simulink model "Stewart"  (Simulink 7.0)
settings: Solver=ode1  StartTime=0.0  StopTime=inf  FixedStep=0.001  RelTol=1e-3
libraries: mblibv1 x50, quarc_library x1
settings Model: Creator=colinlea  LastModifiedBy=colinlea  ExtModeTrigDuration=10000
settings SolverCC: PositivePriorityOrder=on
settings RTWCC: SystemTargetFile=quarc_windows.tlc  TemplateMakefile=quarc_default_tmf  Description=QuaRC Win32 Target  ProcessScript=quarc_windows_make_rtw_hook
settings STFCustomTargetCC: TargetPreCompLibLocation=C:\DOCUME~1\ALLUSE~1\APPLIC~1\QuaRC\lib\2007b\windows\release  GenFloatMathFcnCalls=ANSI_C  SystemTargetFile=quarc_windows.tlc
settings GRTTargetCC: TargetPreCompLibLocation=C:\DOCUME~1\ALLUSE~1\APPLIC~1\QuaRC\lib\2007b\windows\release  CompOptLevelCompliant=off  MatFileLogging=off  ExtMode=on  ExtModeMexFile=quarc_comm
settings SimMechanicsCC: VisOnUpdateDiagram=on  VisDuringSimulation=on

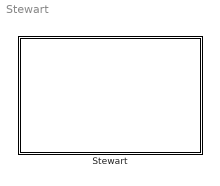
== system Stewart ==
  Stewart : Subsystem

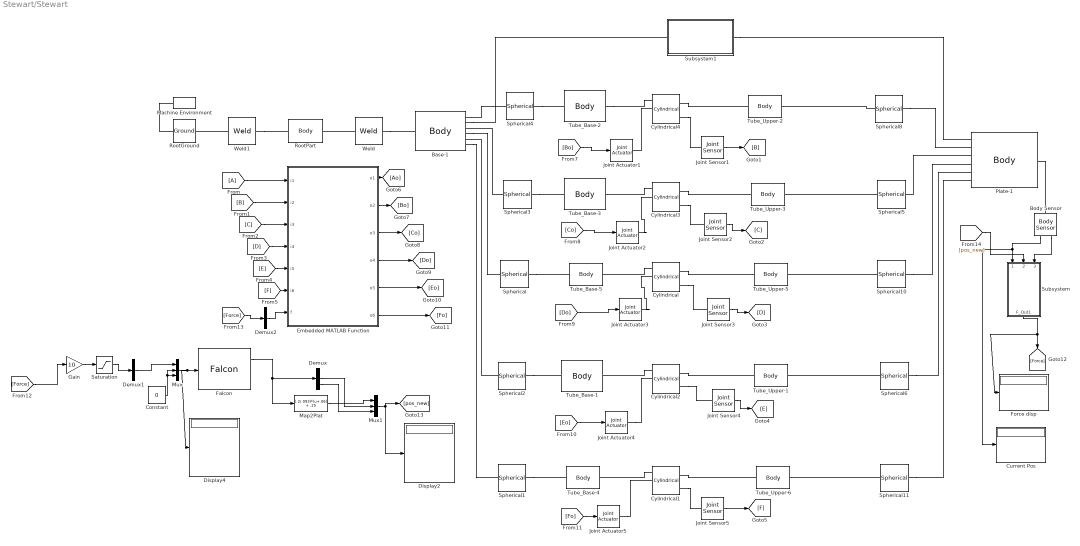
== system Stewart/Stewart ==
  Base-1 : mblibv1/Bodies/Body  DialogController=MECH.DynMechDlgSource  PhysicalDomain=mechanical  SubClassName=Unknown  LeftPortType=workingframe  RightPortType=workingframe  LConnTagsString=CS2  RConnTagsString=CS5|CS8|CS4|CS7|CS3|CS6  DialogClass=MechanicalBodyBlock  Mass=1.0825  MassUnits=kg  InertiaUnits=kg*m^2  Inertia=[0.011284 0 0;0 0.022551 0;0 0 0.011285]  Shape=Cylinder  ShapeDims=[1 1]  ShapeUnits=m  ShapeUse=false  Density=1  DensityUnits=kg/m^3  DensityUse=false  CG=Right$CG$[-0.030204 -0.023928 0.035595]$WORLD$WORLD$m$[1 0 0;0 1 0;0 0 1]$3x3 Transform$rad$WORLD$false  WorkingFrames=Right$CS5$[0.2198 -0.018929 -0.10874]$WORLD$WORLD$m$[1 0 0;0 1 0;0 0 1]$3x3 Transform$rad$WORLD$true#Right$CS8$[0.2198 -0.018929 -0.10874]$WORLD$WORLD$m$[1 0 0;0 1 0;0 0 1]$3x3 Transform$rad$WORLD$true#Left$CS2$[-0.030204 -0.023928 0.035595]$WORLD$WORLD$m$[1 0 0;0 1 0;0 0 1]$3x3 Transform$rad$WORLD$true#Right$CS4$[-0.2802 -0.018929 -0.10874]$WORLD$WORLD$m$[1 0 0;0 1 0;0 0 1]$3x3 Transform$rad$WORLD$true#Right$CS7$[-0.2802 -0.018929 -0.10874]$WORLD$WORLD$m$[1 0 0;0 1 0;0 0 1]$3x3 Transform$rad$WORLD$true#Right$CS3$[-0.030204 -0.018929 0.32426]$WORLD$WORLD$m$[1 0 0;0 1 0;0 0 1]$3x3 Transform$rad$WORLD$true#Right$CS6$[-0.030204 -0.018929 0.32426]$WORLD$WORLD$m$[1 0 0;0 1 0;0 0 1]$3x3 Transform$rad$WORLD$true#Right$CS1$[-0.030204 -0.028928 0.035592]$WORLD$WORLD$m$[1 0 0;0 1 0;0 0 1]$3x3 Transform$rad$WORLD$false  CGPos=[-0.030204 -0.023928 0.035595]  CGRot=[1 0 0;0 1 0;0 0 1]  CS0Pos=[]  CS0Rot=[]  CS1Pos=[-0.030204 -0.028928 0.035592]  CS1Rot=[1 0 0;0 1 0;0 0 1]  CS2Pos=[-0.030204 -0.023928 0.035595]  CS2Rot=[1 0 0;0 1 0;0 0 1]  CS3Pos=[-0.030204 -0.018929 0.32426]  CS3Rot=[1 0 0;0 1 0;0 0 1]  CS4Pos=[-0.2802 -0.018929 -0.10874]  CS4Rot=[1 0 0;0 1 0;0 0 1]  CS5Pos=[0.2198 -0.018929 -0.10874]  CS5Rot=[1 0 0;0 1 0;0 0 1]  CS6Pos=[-0.030204 -0.018929 0.32426]  CS6Rot=[1 0 0;0 1 0;0 0 1]  CS7Pos=[-0.2802 -0.018929 -0.10874]  CS7Rot=[1 0 0;0 1 0;0 0 1]  CS8Pos=[0.2198 -0.018929 -0.10874]  CS8Rot=[1 0 0;0 1 0;0 0 1]  CS9Pos=[]  CS9Rot=[]  CS10Pos=[]  CS10Rot=[]  CS11Pos=[]  CS11Rot=[]  CS12Pos=[]  CS12Rot=[]  CS13Pos=[]  CS13Rot=[]  CS14Pos=[]  CS14Rot=[]  CS15Pos=[]  CS15Rot=[]  CS16Pos=[]  CS16Rot=[]  CS17Pos=[]  CS17Rot=[]  CS18Pos=[]  CS18Rot=[]  CS19Pos=[]  CS19Rot=[]  CS20Pos=[]  CS20Rot=[]
  Body Sensor : mblibv1/Sensors &  Actuators/Body Sensor  Orientation=down  DialogController=MECH.DynMechDlgSource  SystemSampleTime=-1  PhysicalDomain=Mechanical  PortType=blob  Muxed=off  Pose=off  Angle=on  AngleUnits=deg  ArcVelocity=off  ArcVelocityUnits=deg/s  ArcAcceleration=off  ArcAccelerationUnits=deg/s^2  CoordPosition=on  CoordPositionUnits=m  Velocity=on  VelocityUnits=m/s  Acceleration=off  AccelerationUnits=m/s^2  Quaternion=on  QuaternionDT=off  QuaternionDDT=off  QuaternionUnits=off  OutputVector=[1]  ActiveIO=on  Width=6  DialogClass=MechanicalSensorBlock  ReferenceFrame=Absolute (World)
  Constant : Constant  Value=0  OutDataType=sfix(16)  OutScaling=2^0
  Current Pos : Display
  Cylindrical : mblibv1/Joints/Cylindrical  DialogController=MECH.DynMechDlgSource  PhysicalDomain=mechanical  SubClassName=Unknown  LeftPortType=blob  RightPortType=blob  LConnTagsString=__newl0|SA1|SA2  RConnTagsString=__newr0|SA1  NumSAPorts=3  CutJoint=off  MarkAsCut=off  Primitives=prismatic  PrimitiveProps=P1$World$[-0.28308 -0.90664 -0.31285]$prismatic#R1$World$[-0.28308 -0.90664 -0.31285]$revolute  DialogClass=JointBlock  P1Axis=[-0.28308 -0.90664 -0.31285]  R1Axis=[-0.28308 -0.90664 -0.31285]
  Cylindrical1 : mblibv1/Joints/Cylindrical  DialogController=MECH.DynMechDlgSource  PhysicalDomain=mechanical  SubClassName=Unknown  LeftPortType=blob  RightPortType=blob  LConnTagsString=__newl0|SA1|SA2  RConnTagsString=__newr0|SA1  NumSAPorts=3  CutJoint=off  MarkAsCut=off  Primitives=prismatic  PrimitiveProps=P1$World$[0.17265 -0.86638 0.46859]$prismatic#R1$World$[0.17265 -0.86638 0.46859]$revolute  DialogClass=JointBlock  P1Axis=[0.17265 -0.86638 0.46859]  R1Axis=[0.17265 -0.86638 0.46859]
  Cylindrical2 : mblibv1/Joints/Cylindrical  DialogController=MECH.DynMechDlgSource  PhysicalDomain=mechanical  SubClassName=Unknown  LeftPortType=blob  RightPortType=blob  LConnTagsString=__newl0|SA1|SA2  RConnTagsString=__newr0|SA1  NumSAPorts=3  CutJoint=off  MarkAsCut=off  Primitives=prismatic  PrimitiveProps=P1$World$[-0.24223 -0.7709 0.58909]$prismatic#R1$World$[-0.24223 -0.7709 0.58909]$revolute  DialogClass=JointBlock  P1Axis=[-0.24223 -0.7709 0.58909]  R1Axis=[-0.24223 -0.7709 0.58909]
  Cylindrical3 : mblibv1/Joints/Cylindrical  DialogController=MECH.DynMechDlgSource  PhysicalDomain=mechanical  SubClassName=Unknown  LeftPortType=blob  RightPortType=blob  LConnTagsString=__newl0|SA1|SA2  RConnTagsString=__newr0|SA1  NumSAPorts=3  CutJoint=off  MarkAsCut=off  Primitives=prismatic  PrimitiveProps=P1$World$[-0.42557 -0.8936 0.14272]$prismatic#R1$World$[-0.42557 -0.8936 0.14272]$revolute  DialogClass=JointBlock  P1Axis=[-0.42557 -0.8936 0.14272]  R1Axis=[-0.42557 -0.8936 0.14272]
  Cylindrical4 : mblibv1/Joints/Cylindrical  DialogController=MECH.DynMechDlgSource  PhysicalDomain=mechanical  SubClassName=Unknown  LeftPortType=blob  RightPortType=blob  LConnTagsString=__newl0|SA1|SA2  RConnTagsString=__newr0|SA1  NumSAPorts=3  CutJoint=off  MarkAsCut=off  Primitives=prismatic  PrimitiveProps=P1$World$[0.24469 -0.94526 -0.21591]$prismatic#R1$World$[0.24469 -0.94526 -0.21591]$revolute  DialogClass=JointBlock  P1Axis=[0.24469 -0.94526 -0.21591]  R1Axis=[0.24469 -0.94526 -0.21591]
  Demux : Demux  Outputs=3
  Demux1 : Demux  Outputs=3
  Demux2 : Demux  Outputs=3
  Display2 : Display
  Display4 : Display
  Embedded MATLAB Function : Stateflow chart
  Falcon : quarc_library/Devices/Third-Party/Novint/Falcon  sample_time=qc_get_step_size  show_calibrate=off
  Force disp : Display
  Gain : Gain  Gain=10  ParameterDataType=sfix(16)  ParameterScaling=2^0  OutDataType=sfix(16)  OutScaling=2^0
  Joint Actuator{1..5} (5 alike) : mblibv1/Sensors &  Actuators/Joint Actuator  DialogController=MECH.DynMechDlgSource  SystemSampleTime=-1  PhysicalDomain=Mechanical  PortType=blob  ActuationStyle=Force  AngleUnits=deg  ArcVelocityUnits=deg/s  ArcAccelerationUnits=deg/s^2  CoordPositionUnits=m  VelocityUnits=m/s  AccelerationUnits=m/s^2  ForceUnits=N  TorqueUnits=N*m  ActiveIO=on  Width=1  DialogClass=MechanicalActuatorBlock  Primitive=P1  ReferenceFrame=Absolute (World)
  Joint Sensor{1..5} (5 alike) : mblibv1/Sensors &  Actuators/Joint Sensor  DialogController=MECH.DynMechDlgSource  SystemSampleTime=-1  PhysicalDomain=Mechanical  PortType=blob  Muxed=on  Pose=off  Angle=on  AngleUnits=deg  ArcVelocity=off  ArcVelocityUnits=deg/s  ArcAcceleration=off  ArcAccelerationUnits=deg/s^2  CoordPosition=on  CoordPositionUnits=m  Velocity=off  VelocityUnits=m/s  Acceleration=off  AccelerationUnits=m/s^2  Quaternion=on  QuaternionDT=off  QuaternionDDT=off  QuaternionUnits=off  OutputVector=[1]  ActiveIO=on  Width=1  DialogClass=MechanicalSensorBlock  Primitive=P1  Force=off  ForceUnits=N  Torque=off  TorqueUnits=N-m  ReferenceFrame=Absolute (World)  ReactionSensedSide=Base  ReactionReferenceFrame=Absolute (World)  ReactionForce=off  ReactionForceUnits=N  ReactionMoment=off  ReactionMomentUnits=N-m
  Machine Environment : mblibv1/Bodies/Machine Environment  Orientation=left  DialogController=MECH.DialogSource  SystemSampleTime=-1  PortType=env  PhysicalDomain=Mechanical  DialogTemplateClass=MECH.MachineEnvironment  SyncWhenCopied=off  Gravity=[0 0 0]  GravityUnits=m/s^2  GravityAsSignal=off  Dimensionality=Auto-detect  AnalysisType=Forward dynamics  LinearAssemblyTolerance=1e-3  LinearAssemblyToleranceUnits=m  AngularAssemblyTolerance=1e-3  AngularAssemblyToleranceUnits=rad  ConstraintSolverType=Stabilizing  ConstraintRelTolerance=1e-4  ConstraintAbsTolerance=1e-4  UseRobustSingularityHandling=off  RedundancyAnalysisToleranceType=Automatically select tolerance  RedundancyAnalysisTolerance=1e-14  StatePerturbationType=Fixed  PerturbationSize=1e-5  VisualizeMachine=on
  Map2Plat : Fcn  Expr=(.2/.093)*(u+.06) + .25
  Mux : Mux  Inputs=3
  Mux1 : Mux  Inputs=3
  Plate-1 : mblibv1/Bodies/Body  DialogController=MECH.DynMechDlgSource  PhysicalDomain=mechanical  SubClassName=Unknown  LeftPortType=workingframe  RightPortType=workingframe  LConnTagsString=CS5|CS4|CS2|CS6|CS3|CS7  RConnTagsString=CG  DialogClass=MechanicalBodyBlock  Mass=0.27063  MassUnits=kg  InertiaUnits=kg*m^2  Inertia=[0.00070697 0 0;0 0.0014095 0;0 0 0.00070701]  Shape=Cylinder  ShapeDims=[1 1]  ShapeUnits=m  ShapeUse=false  Density=1  DensityUnits=kg/m^3  DensityUse=false  CG=Right$CG$[-0.032335 0.43541 -0.043031]$WORLD$WORLD$m$[0.19654 0.14624 0.96953;-0.26061 0.96104 -0.092126;-0.94523 -0.23456 0.227]$3x3 Transform$rad$WORLD$true  WorkingFrames=Left$CS5$[-0.078466 0.40468 -0.17639]$WORLD$WORLD$m$[1 0 0;0 1 0;0 0 1]$3x3 Transform$rad$WORLD$true#Left$CS4$[0.10687 0.41731 -0.0090952]$WORLD$WORLD$m$[1 0 0;0 1 0;0 0 1]$3x3 Transform$rad$WORLD$true#Left$CS2$[-0.078466 0.40468 -0.17639]$WORLD$WORLD$m$[1 0 0;0 1 0;0 0 1]$3x3 Transform$rad$WORLD$true#Left$CS6$[-0.1276 0.46983 0.059914]$WORLD$WORLD$m$[1 0 0;0 1 0;0 0 1]$3x3 Transform$rad$WORLD$true#Left$CS3$[0.10687 0.41731 -0.0090952]$WORLD$WORLD$m$[1 0 0;0 1 0;0 0 1]$3x3 Transform$rad$WORLD$true#Left$CS7$[-0.1276 0.46983 0.059914]$WORLD$WORLD$m$[1 0 0;0 1 0;0 0 1]$3x3 Transform$rad$WORLD$true#Right$CS1$[-0.033072 0.43061 -0.04186]$WORLD$WORLD$m$[0.19654 0.14624 0.96953;-0.26061 0.96104 -0.092126;-0.94523 -0.23456 0.227]$3x3 Transform$rad$WORLD$false  CGPos=[-0.032335 0.43541 -0.043031]  CGRot=[0.19654 0.14624 0.96953;-0.26061 0.96104 -0.092126;-0.94523 -0.23456 0.227]  CS0Pos=[]  CS0Rot=[]  CS1Pos=[-0.033072 0.43061 -0.04186]  CS1Rot=[0.19654 0.14624 0.96953;-0.26061 0.96104 -0.092126;-0.94523 -0.23456 0.227]  CS2Pos=[-0.078466 0.40468 -0.17639]  CS2Rot=[1 0 0;0 1 0;0 0 1]  CS3Pos=[0.10687 0.41731 -0.0090952]  CS3Rot=[1 0 0;0 1 0;0 0 1]  CS4Pos=[0.10687 0.41731 -0.0090952]  CS4Rot=[1 0 0;0 1 0;0 0 1]  CS5Pos=[-0.078466 0.40468 -0.17639]  CS5Rot=[1 0 0;0 1 0;0 0 1]  CS6Pos=[-0.1276 0.46983 0.059914]  CS6Rot=[1 0 0;0 1 0;0 0 1]  CS7Pos=[-0.1276 0.46983 0.059914]  CS7Rot=[1 0 0;0 1 0;0 0 1]  CS8Pos=[]  CS8Rot=[]  CS9Pos=[]  CS9Rot=[]  CS10Pos=[]  CS10Rot=[]  CS11Pos=[]  CS11Rot=[]  CS12Pos=[]  CS12Rot=[]  CS13Pos=[]  CS13Rot=[]  CS14Pos=[]  CS14Rot=[]  CS15Pos=[]  CS15Rot=[]  CS16Pos=[]  CS16Rot=[]  CS17Pos=[]  CS17Rot=[]  CS18Pos=[]  CS18Rot=[]  CS19Pos=[]  CS19Rot=[]  CS20Pos=[]  CS20Rot=[]
  RootGround : mblibv1/Bodies/Ground  DialogController=MECH.DynMechDlgSource  SystemSampleTime=-1  LeftPortType=env  RightPortType=workingframe  PhysicalDomain=Mechanical  DialogClass=GroundBlock  CoordPosition=[-0.031154 0.13602 0.0091958]  CoordPositionUnits=m  StateVectorMgrId=0  MachineId=[0 0]  ShowEnvPort=on
  RootPart : mblibv1/Bodies/Body  DialogController=MECH.DynMechDlgSource  PhysicalDomain=mechanical  SubClassName=Unknown  LeftPortType=workingframe  RightPortType=workingframe  LConnTagsString=CS3  RConnTagsString=CS2  DialogClass=MechanicalBodyBlock  Mass=0  MassUnits=kg  InertiaUnits=kg*m^2  Inertia=[0 0 0;0 0 0;0 0 0]  Shape=Cylinder  ShapeDims=[1 1]  ShapeUnits=m  ShapeUse=false  Density=1  DensityUnits=kg/m^3  DensityUse=false  CG=Right$CG$[-0.031154 0.13602 0.0091958]$WORLD$WORLD$m$[1 0 0;0 1 0;0 0 1]$3x3 Transform$rad$WORLD$  WorkingFrames=Right$CS2$[-0.030204 -0.023928 0.035595]$WORLD$WORLD$m$[1 0 0;0 1 0;0 0 1]$3x3 Transform$rad$WORLD$true#Left$CS3$[-0.031154 0.13602 0.0091958]$WORLD$WORLD$m$[1 0 0;0 1 0;0 0 1]$3x3 Transform$rad$WORLD$true#Right$CS1$[0 0 0]$WORLD$WORLD$m$[1 0 0;0 1 0;0 0 1]$3x3 Transform$rad$WORLD$  CGPos=[-0.031154 0.13602 0.0091958]  CGRot=[1 0 0;0 1 0;0 0 1]  CS0Pos=[]  CS0Rot=[]  CS1Pos=[0 0 0]  CS1Rot=[1 0 0;0 1 0;0 0 1]  CS2Pos=[-0.030204 -0.023928 0.035595]  CS2Rot=[1 0 0;0 1 0;0 0 1]  CS3Pos=[-0.031154 0.13602 0.0091958]  CS3Rot=[1 0 0;0 1 0;0 0 1]  CS4Pos=[]  CS4Rot=[]  CS5Pos=[]  CS5Rot=[]  CS6Pos=[]  CS6Rot=[]  CS7Pos=[]  CS7Rot=[]  CS8Pos=[]  CS8Rot=[]  CS9Pos=[]  CS9Rot=[]  CS10Pos=[]  CS10Rot=[]  CS11Pos=[]  CS11Rot=[]  CS12Pos=[]  CS12Rot=[]  CS13Pos=[]  CS13Rot=[]  CS14Pos=[]  CS14Rot=[]  CS15Pos=[]  CS15Rot=[]  CS16Pos=[]  CS16Rot=[]  CS17Pos=[]  CS17Rot=[]  CS18Pos=[]  CS18Rot=[]  CS19Pos=[]  CS19Rot=[]  CS20Pos=[]  CS20Rot=[]
  Saturation : Saturate  UpperLimit=9  LowerLimit=-9  OutDataType=sfix(16)  OutScaling=2^0
  Spherical{,1..6,8,10..11} (10 alike) : mblibv1/Joints/Spherical  DialogController=MECH.DynMechDlgSource  PhysicalDomain=mechanical  SubClassName=Unknown  LeftPortType=blob  RightPortType=blob  LConnTagsString=__newl0  RConnTagsString=__newr0  NumSAPorts=0  CutJoint=off  MarkAsCut=off  Primitives=spherical  PrimitiveProps=S$WORLD$[0 0 0]$spherical  DialogClass=JointBlock  SAxis=[0 0 0]
  Subsystem : Subsystem  Orientation=down
  Subsystem1 : Subsystem
  Tube_Base-1 : mblibv1/Bodies/Body  DialogController=MECH.DynMechDlgSource  PhysicalDomain=mechanical  SubClassName=Unknown  LeftPortType=workingframe  RightPortType=workingframe  LConnTagsString=CS3  RConnTagsString=CS4  DialogClass=MechanicalBodyBlock  Mass=0.12566  MassUnits=kg  InertiaUnits=kg*m^2  Inertia=[0.0016787 0 0;0 6.2832e-006 0;0 0 0.0016787]  Shape=Cylinder  ShapeDims=[1 1]  ShapeUnits=m  ShapeUse=false  Density=1  DensityUnits=kg/m^3  DensityUse=false  CG=Right$CG$[0.018242 0.13525 0.20644]$WORLD$WORLD$m$[0.96834 0.24223 0.060313;-0.22984 0.7709 0.59404;0.097398 -0.58909 0.80217]$3x3 Transform$rad$WORLD$false  WorkingFrames=Left$CS3$[-0.030204 -0.018929 0.32426]$WORLD$WORLD$m$[1 0 0;0 1 0;0 0 1]$3x3 Transform$rad$WORLD$true#Right$CS4$[0.066688 0.28943 0.088624]$WORLD$WORLD$m$[1 0 0;0 1 0;0 0 1]$3x3 Transform$rad$WORLD$true#Right$CS2$[-0.030204 -0.018929 0.32426]$WORLD$WORLD$m$[1 0 0;0 1 0;0 0 1]$3x3 Transform$rad$WORLD$false#Right$CS1$[-0.030204 -0.018929 0.32426]$WORLD$WORLD$m$[0.96834 0.24223 0.060313;-0.22984 0.7709 0.59404;0.097398 -0.58909 0.80217]$3x3 Transform$rad$WORLD$false  CGPos=[0.018242 0.13525 0.20644]  CGRot=[0.96834 0.24223 0.060313;-0.22984 0.7709 0.59404;0.097398 -0.58909 0.80217]  CS0Pos=[]  CS0Rot=[]  CS1Pos=[-0.030204 -0.018929 0.32426]  CS1Rot=[0.96834 0.24223 0.060313;-0.22984 0.7709 0.59404;0.097398 -0.58909 0.80217]  CS2Pos=[-0.030204 -0.018929 0.32426]  CS2Rot=[1 0 0;0 1 0;0 0 1]  CS3Pos=[-0.030204 -0.018929 0.32426]  CS3Rot=[1 0 0;0 1 0;0 0 1]  CS4Pos=[0.066688 0.28943 0.088624]  CS4Rot=[1 0 0;0 1 0;0 0 1]  CS5Pos=[]  CS5Rot=[]  CS6Pos=[]  CS6Rot=[]  CS7Pos=[]  CS7Rot=[]  CS8Pos=[]  CS8Rot=[]  CS9Pos=[]  CS9Rot=[]  CS10Pos=[]  CS10Rot=[]  CS11Pos=[]  CS11Rot=[]  CS12Pos=[]  CS12Rot=[]  CS13Pos=[]  CS13Rot=[]  CS14Pos=[]  CS14Rot=[]  CS15Pos=[]  CS15Rot=[]  CS16Pos=[]  CS16Rot=[]  CS17Pos=[]  CS17Rot=[]  CS18Pos=[]  CS18Rot=[]  CS19Pos=[]  CS19Rot=[]  CS20Pos=[]  CS20Rot=[]
  Tube_Base-2 : mblibv1/Bodies/Body  DialogController=MECH.DynMechDlgSource  PhysicalDomain=mechanical  SubClassName=Unknown  LeftPortType=workingframe  RightPortType=workingframe  LConnTagsString=CS2  RConnTagsString=CS3  DialogClass=MechanicalBodyBlock  Mass=0.12566  MassUnits=kg  InertiaUnits=kg*m^2  Inertia=[0.0016787 0 0;0 6.2832e-006 0;0 0 0.0016787]  Shape=Cylinder  ShapeDims=[1 1]  ShapeUnits=m  ShapeUse=false  Density=1  DensityUnits=kg/m^3  DensityUse=false  CG=Right$CG$[0.17086 0.17012 -0.065556]$WORLD$WORLD$m$[0.96619 -0.24469 0.081267;0.25637 0.94526 -0.2019;-0.027415 0.21591 0.97603]$3x3 Transform$rad$WORLD$false  WorkingFrames=Right$CS4$[0.2198 -0.018929 -0.10874]$WORLD$WORLD$m$[1 0 0;0 1 0;0 0 1]$3x3 Transform$rad$WORLD$false#Right$CS3$[0.12192 0.35917 -0.022374]$WORLD$WORLD$m$[1 0 0;0 1 0;0 0 1]$3x3 Transform$rad$WORLD$true#Left$CS2$[0.2198 -0.018929 -0.10874]$WORLD$WORLD$m$[1 0 0;0 1 0;0 0 1]$3x3 Transform$rad$WORLD$true#Right$CS1$[0.2198 -0.018929 -0.10874]$WORLD$WORLD$m$[0.96619 -0.24469 0.081267;0.25637 0.94526 -0.2019;-0.027415 0.21591 0.97603]$3x3 Transform$rad$WORLD$false  CGPos=[0.17086 0.17012 -0.065556]  CGRot=[0.96619 -0.24469 0.081267;0.25637 0.94526 -0.2019;-0.027415 0.21591 0.97603]  CS0Pos=[]  CS0Rot=[]  CS1Pos=[0.2198 -0.018929 -0.10874]  CS1Rot=[0.96619 -0.24469 0.081267;0.25637 0.94526 -0.2019;-0.027415 0.21591 0.97603]  CS2Pos=[0.2198 -0.018929 -0.10874]  CS2Rot=[1 0 0;0 1 0;0 0 1]  CS3Pos=[0.12192 0.35917 -0.022374]  CS3Rot=[1 0 0;0 1 0;0 0 1]  CS4Pos=[0.2198 -0.018929 -0.10874]  CS4Rot=[1 0 0;0 1 0;0 0 1]  CS5Pos=[]  CS5Rot=[]  CS6Pos=[]  CS6Rot=[]  CS7Pos=[]  CS7Rot=[]  CS8Pos=[]  CS8Rot=[]  CS9Pos=[]  CS9Rot=[]  CS10Pos=[]  CS10Rot=[]  CS11Pos=[]  CS11Rot=[]  CS12Pos=[]  CS12Rot=[]  CS13Pos=[]  CS13Rot=[]  CS14Pos=[]  CS14Rot=[]  CS15Pos=[]  CS15Rot=[]  CS16Pos=[]  CS16Rot=[]  CS17Pos=[]  CS17Rot=[]  CS18Pos=[]  CS18Rot=[]  CS19Pos=[]  CS19Rot=[]  CS20Pos=[]  CS20Rot=[]
  Tube_Base-3 : mblibv1/Bodies/Body  DialogController=MECH.DynMechDlgSource  PhysicalDomain=mechanical  SubClassName=Unknown  LeftPortType=workingframe  RightPortType=workingframe  LConnTagsString=CS3  RConnTagsString=CS4  DialogClass=MechanicalBodyBlock  Mass=0.12566  MassUnits=kg  InertiaUnits=kg*m^2  Inertia=[0.0016787 0 0;0 6.2832e-006 0;0 0 0.0016787]  Shape=Cylinder  ShapeDims=[1 1]  ShapeUnits=m  ShapeUse=false  Density=1  DensityUnits=kg/m^3  DensityUse=false  CG=Right$CG$[-0.19509 0.15979 -0.13728]$WORLD$WORLD$m$[0.9049 0.42557 -0.0073951;-0.41894 0.8936 0.16114;0.075184 -0.14272 0.9869]$3x3 Transform$rad$WORLD$false  WorkingFrames=Right$CS4$[-0.10998 0.33851 -0.16583]$WORLD$WORLD$m$[1 0 0;0 1 0;0 0 1]$3x3 Transform$rad$WORLD$true#Left$CS3$[-0.2802 -0.018929 -0.10874]$WORLD$WORLD$m$[1 0 0;0 1 0;0 0 1]$3x3 Transform$rad$WORLD$true#Right$CS2$[-0.2802 -0.018929 -0.10874]$WORLD$WORLD$m$[1 0 0;0 1 0;0 0 1]$3x3 Transform$rad$WORLD$false#Right$CS1$[-0.2802 -0.018929 -0.10874]$WORLD$WORLD$m$[0.9049 0.42557 -0.0073951;-0.41894 0.8936 0.16114;0.075184 -0.14272 0.9869]$3x3 Transform$rad$WORLD$false  CGPos=[-0.19509 0.15979 -0.13728]  CGRot=[0.9049 0.42557 -0.0073951;-0.41894 0.8936 0.16114;0.075184 -0.14272 0.9869]  CS0Pos=[]  CS0Rot=[]  CS1Pos=[-0.2802 -0.018929 -0.10874]  CS1Rot=[0.9049 0.42557 -0.0073951;-0.41894 0.8936 0.16114;0.075184 -0.14272 0.9869]  CS2Pos=[-0.2802 -0.018929 -0.10874]  CS2Rot=[1 0 0;0 1 0;0 0 1]  CS3Pos=[-0.2802 -0.018929 -0.10874]  CS3Rot=[1 0 0;0 1 0;0 0 1]  CS4Pos=[-0.10998 0.33851 -0.16583]  CS4Rot=[1 0 0;0 1 0;0 0 1]  CS5Pos=[]  CS5Rot=[]  CS6Pos=[]  CS6Rot=[]  CS7Pos=[]  CS7Rot=[]  CS8Pos=[]  CS8Rot=[]  CS9Pos=[]  CS9Rot=[]  CS10Pos=[]  CS10Rot=[]  CS11Pos=[]  CS11Rot=[]  CS12Pos=[]  CS12Rot=[]  CS13Pos=[]  CS13Rot=[]  CS14Pos=[]  CS14Rot=[]  CS15Pos=[]  CS15Rot=[]  CS16Pos=[]  CS16Rot=[]  CS17Pos=[]  CS17Rot=[]  CS18Pos=[]  CS18Rot=[]  CS19Pos=[]  CS19Rot=[]  CS20Pos=[]  CS20Rot=[]
  Tube_Base-4 : mblibv1/Bodies/Body  DialogController=MECH.DynMechDlgSource  PhysicalDomain=mechanical  SubClassName=Unknown  LeftPortType=workingframe  RightPortType=workingframe  LConnTagsString=CS2  RConnTagsString=CS3  DialogClass=MechanicalBodyBlock  Mass=0.12566  MassUnits=kg  InertiaUnits=kg*m^2  Inertia=[0.0016787 0 0;0 6.2832e-006 0;0 0 0.0016787]  Shape=Cylinder  ShapeDims=[1 1]  ShapeUnits=m  ShapeUse=false  Density=1  DensityUnits=kg/m^3  DensityUse=false  CG=Right$CG$[-0.064733 0.15435 0.23054]$WORLD$WORLD$m$[0.98497 -0.17265 -0.0047879;0.15417 0.86638 0.47499;-0.077857 -0.46859 0.87998]$3x3 Transform$rad$WORLD$  WorkingFrames=Right$CS3$[-0.099263 0.32763 0.13683]$WORLD$WORLD$m$[1 0 0;0 1 0;0 0 1]$3x3 Transform$rad$WORLD$true#Left$CS2$[-0.030204 -0.018929 0.32426]$WORLD$WORLD$m$[1 0 0;0 1 0;0 0 1]$3x3 Transform$rad$WORLD$true#Right$CS1$[-0.030204 -0.018929 0.32426]$WORLD$WORLD$m$[0.98497 -0.17265 -0.0047879;0.15417 0.86638 0.47499;-0.077857 -0.46859 0.87998]$3x3 Transform$rad$WORLD$  CGPos=[-0.064733 0.15435 0.23054]  CGRot=[0.98497 -0.17265 -0.0047879;0.15417 0.86638 0.47499;-0.077857 -0.46859 0.87998]  CS0Pos=[]  CS0Rot=[]  CS1Pos=[-0.030204 -0.018929 0.32426]  CS1Rot=[0.98497 -0.17265 -0.0047879;0.15417 0.86638 0.47499;-0.077857 -0.46859 0.87998]  CS2Pos=[-0.030204 -0.018929 0.32426]  CS2Rot=[1 0 0;0 1 0;0 0 1]  CS3Pos=[-0.099263 0.32763 0.13683]  CS3Rot=[1 0 0;0 1 0;0 0 1]  CS4Pos=[]  CS4Rot=[]  CS5Pos=[]  CS5Rot=[]  CS6Pos=[]  CS6Rot=[]  CS7Pos=[]  CS7Rot=[]  CS8Pos=[]  CS8Rot=[]  CS9Pos=[]  CS9Rot=[]  CS10Pos=[]  CS10Rot=[]  CS11Pos=[]  CS11Rot=[]  CS12Pos=[]  CS12Rot=[]  CS13Pos=[]  CS13Rot=[]  CS14Pos=[]  CS14Rot=[]  CS15Pos=[]  CS15Rot=[]  CS16Pos=[]  CS16Rot=[]  CS17Pos=[]  CS17Rot=[]  CS18Pos=[]  CS18Rot=[]  CS19Pos=[]  CS19Rot=[]  CS20Pos=[]  CS20Rot=[]
  Tube_Base-5 : mblibv1/Bodies/Body  DialogController=MECH.DynMechDlgSource  PhysicalDomain=mechanical  SubClassName=Unknown  LeftPortType=workingframe  RightPortType=workingframe  LConnTagsString=CS2  RConnTagsString=CS3  DialogClass=MechanicalBodyBlock  Mass=0.12566  MassUnits=kg  InertiaUnits=kg*m^2  Inertia=[0.0016787 0 0;0 6.2832e-006 0;0 0 0.0016787]  Shape=Cylinder  ShapeDims=[1 1]  ShapeUnits=m  ShapeUse=false  Density=1  DensityUnits=kg/m^3  DensityUse=false  CG=Right$CG$[-0.22359 0.1624 -0.046169]$WORLD$WORLD$m$[0.95908 0.28308 0.0054982;-0.26572 0.90664 -0.32772;-0.097753 0.31284 0.94476]$3x3 Transform$rad$WORLD$  WorkingFrames=Left$CS2$[-0.2802 -0.018929 -0.10874]$WORLD$WORLD$m$[1 0 0;0 1 0;0 0 1]$3x3 Transform$rad$WORLD$true#Right$CS3$[-0.16697 0.34373 0.0164]$WORLD$WORLD$m$[1 0 0;0 1 0;0 0 1]$3x3 Transform$rad$WORLD$true#Right$CS1$[-0.2802 -0.018929 -0.10874]$WORLD$WORLD$m$[0.95908 0.28308 0.0054982;-0.26572 0.90664 -0.32772;-0.097753 0.31284 0.94476]$3x3 Transform$rad$WORLD$  CGPos=[-0.22359 0.1624 -0.046169]  CGRot=[0.95908 0.28308 0.0054982;-0.26572 0.90664 -0.32772;-0.097753 0.31284 0.94476]  CS0Pos=[]  CS0Rot=[]  CS1Pos=[-0.2802 -0.018929 -0.10874]  CS1Rot=[0.95908 0.28308 0.0054982;-0.26572 0.90664 -0.32772;-0.097753 0.31284 0.94476]  CS2Pos=[-0.2802 -0.018929 -0.10874]  CS2Rot=[1 0 0;0 1 0;0 0 1]  CS3Pos=[-0.16697 0.34373 0.0164]  CS3Rot=[1 0 0;0 1 0;0 0 1]  CS4Pos=[]  CS4Rot=[]  CS5Pos=[]  CS5Rot=[]  CS6Pos=[]  CS6Rot=[]  CS7Pos=[]  CS7Rot=[]  CS8Pos=[]  CS8Rot=[]  CS9Pos=[]  CS9Rot=[]  CS10Pos=[]  CS10Rot=[]  CS11Pos=[]  CS11Rot=[]  CS12Pos=[]  CS12Rot=[]  CS13Pos=[]  CS13Rot=[]  CS14Pos=[]  CS14Rot=[]  CS15Pos=[]  CS15Rot=[]  CS16Pos=[]  CS16Rot=[]  CS17Pos=[]  CS17Rot=[]  CS18Pos=[]  CS18Rot=[]  CS19Pos=[]  CS19Rot=[]  CS20Pos=[]  CS20Rot=[]
  Tube_Upper-1 : mblibv1/Bodies/Body  DialogController=MECH.DynMechDlgSource  PhysicalDomain=mechanical  SubClassName=Unknown  LeftPortType=workingframe  RightPortType=workingframe  LConnTagsString=CS2  RConnTagsString=CS3  DialogClass=MechanicalBodyBlock  Mass=0.062832  MassUnits=kg  InertiaUnits=kg*m^2  Inertia=[0.00021101 0 0;0 3.1416e-006 0;0 0 0.00021101]  Shape=Cylinder  ShapeDims=[1 1]  ShapeUnits=m  ShapeUse=false  Density=1  DensityUnits=kg/m^3  DensityUse=false  CG=Right$CG$[0.082647 0.34022 0.049814]$WORLD$WORLD$m$[-0.92846 0.24223 0.28158;0.0079695 0.7709 -0.6369;-0.37135 -0.58909 -0.71768]$3x3 Transform$rad$WORLD$  WorkingFrames=Right$CS3$[0.10687 0.41731 -0.0090952]$WORLD$WORLD$m$[1 0 0;0 1 0;0 0 1]$3x3 Transform$rad$WORLD$true#Left$CS2$[0.066688 0.28943 0.088624]$WORLD$WORLD$m$[1 0 0;0 1 0;0 0 1]$3x3 Transform$rad$WORLD$true#Right$CS1$[0.058424 0.26313 0.10872]$WORLD$WORLD$m$[-0.92846 0.24223 0.28158;0.0079695 0.7709 -0.6369;-0.37135 -0.58909 -0.71768]$3x3 Transform$rad$WORLD$  CGPos=[0.082647 0.34022 0.049814]  CGRot=[-0.92846 0.24223 0.28158;0.0079695 0.7709 -0.6369;-0.37135 -0.58909 -0.71768]  CS0Pos=[]  CS0Rot=[]  CS1Pos=[0.058424 0.26313 0.10872]  CS1Rot=[-0.92846 0.24223 0.28158;0.0079695 0.7709 -0.6369;-0.37135 -0.58909 -0.71768]  CS2Pos=[0.066688 0.28943 0.088624]  CS2Rot=[1 0 0;0 1 0;0 0 1]  CS3Pos=[0.10687 0.41731 -0.0090952]  CS3Rot=[1 0 0;0 1 0;0 0 1]  CS4Pos=[]  CS4Rot=[]  CS5Pos=[]  CS5Rot=[]  CS6Pos=[]  CS6Rot=[]  CS7Pos=[]  CS7Rot=[]  CS8Pos=[]  CS8Rot=[]  CS9Pos=[]  CS9Rot=[]  CS10Pos=[]  CS10Rot=[]  CS11Pos=[]  CS11Rot=[]  CS12Pos=[]  CS12Rot=[]  CS13Pos=[]  CS13Rot=[]  CS14Pos=[]  CS14Rot=[]  CS15Pos=[]  CS15Rot=[]  CS16Pos=[]  CS16Rot=[]  CS17Pos=[]  CS17Rot=[]  CS18Pos=[]  CS18Rot=[]  CS19Pos=[]  CS19Rot=[]  CS20Pos=[]  CS20Rot=[]
  Tube_Upper-2 : mblibv1/Bodies/Body  DialogController=MECH.DynMechDlgSource  PhysicalDomain=mechanical  SubClassName=Unknown  LeftPortType=workingframe  RightPortType=workingframe  LConnTagsString=CS2  RConnTagsString=CS3  DialogClass=MechanicalBodyBlock  Mass=0.062832  MassUnits=kg  InertiaUnits=kg*m^2  Inertia=[0.00021101 0 0;0 3.1416e-006 0;0 0 0.00021101]  Shape=Cylinder  ShapeDims=[1 1]  ShapeUnits=m  ShapeUse=false  Density=1  DensityUnits=kg/m^3  DensityUse=false  CG=Right$CG$[0.13134 0.32278 -0.030686]$WORLD$WORLD$m$[-0.15975 -0.24469 -0.95635;-0.25894 0.94526 -0.1986;0.95259 0.21591 -0.21436]$3x3 Transform$rad$WORLD$  WorkingFrames=Right$CS3$[0.10687 0.41731 -0.0090952]$WORLD$WORLD$m$[1 0 0;0 1 0;0 0 1]$3x3 Transform$rad$WORLD$true#Left$CS2$[0.12192 0.35917 -0.022374]$WORLD$WORLD$m$[1 0 0;0 1 0;0 0 1]$3x3 Transform$rad$WORLD$true#Right$CS1$[0.15581 0.22826 -0.052277]$WORLD$WORLD$m$[-0.15975 -0.24469 -0.95635;-0.25894 0.94526 -0.1986;0.95259 0.21591 -0.21436]$3x3 Transform$rad$WORLD$  CGPos=[0.13134 0.32278 -0.030686]  CGRot=[-0.15975 -0.24469 -0.95635;-0.25894 0.94526 -0.1986;0.95259 0.21591 -0.21436]  CS0Pos=[]  CS0Rot=[]  CS1Pos=[0.15581 0.22826 -0.052277]  CS1Rot=[-0.15975 -0.24469 -0.95635;-0.25894 0.94526 -0.1986;0.95259 0.21591 -0.21436]  CS2Pos=[0.12192 0.35917 -0.022374]  CS2Rot=[1 0 0;0 1 0;0 0 1]  CS3Pos=[0.10687 0.41731 -0.0090952]  CS3Rot=[1 0 0;0 1 0;0 0 1]  CS4Pos=[]  CS4Rot=[]  CS5Pos=[]  CS5Rot=[]  CS6Pos=[]  CS6Rot=[]  CS7Pos=[]  CS7Rot=[]  CS8Pos=[]  CS8Rot=[]  CS9Pos=[]  CS9Rot=[]  CS10Pos=[]  CS10Rot=[]  CS11Pos=[]  CS11Rot=[]  CS12Pos=[]  CS12Rot=[]  CS13Pos=[]  CS13Rot=[]  CS14Pos=[]  CS14Rot=[]  CS15Pos=[]  CS15Rot=[]  CS16Pos=[]  CS16Rot=[]  CS17Pos=[]  CS17Rot=[]  CS18Pos=[]  CS18Rot=[]  CS19Pos=[]  CS19Rot=[]  CS20Pos=[]  CS20Rot=[]
  Tube_Upper-3 : mblibv1/Bodies/Body  DialogController=MECH.DynMechDlgSource  PhysicalDomain=mechanical  SubClassName=Unknown  LeftPortType=workingframe  RightPortType=workingframe  LConnTagsString=CS2  RConnTagsString=CS3  DialogClass=MechanicalBodyBlock  Mass=0.062832  MassUnits=kg  InertiaUnits=kg*m^2  Inertia=[0.00021101 0 0;0 3.1416e-006 0;0 0 0.00021101]  Shape=Cylinder  ShapeDims=[1 1]  ShapeUnits=m  ShapeUse=false  Density=1  DensityUnits=kg/m^3  DensityUse=false  CG=Right$CG$[-0.12102 0.31532 -0.16212]$WORLD$WORLD$m$[0.57849 0.42557 -0.69587;-0.14737 0.8936 0.42398;0.80226 -0.14272 0.57966]$3x3 Transform$rad$WORLD$  WorkingFrames=Left$CS2$[-0.10998 0.33851 -0.16583]$WORLD$WORLD$m$[1 0 0;0 1 0;0 0 1]$3x3 Transform$rad$WORLD$true#Right$CS3$[-0.078466 0.40468 -0.17639]$WORLD$WORLD$m$[1 0 0;0 1 0;0 0 1]$3x3 Transform$rad$WORLD$true#Right$CS1$[-0.16358 0.22596 -0.14785]$WORLD$WORLD$m$[0.57849 0.42557 -0.69587;-0.14737 0.8936 0.42398;0.80226 -0.14272 0.57966]$3x3 Transform$rad$WORLD$  CGPos=[-0.12102 0.31532 -0.16212]  CGRot=[0.57849 0.42557 -0.69587;-0.14737 0.8936 0.42398;0.80226 -0.14272 0.57966]  CS0Pos=[]  CS0Rot=[]  CS1Pos=[-0.16358 0.22596 -0.14785]  CS1Rot=[0.57849 0.42557 -0.69587;-0.14737 0.8936 0.42398;0.80226 -0.14272 0.57966]  CS2Pos=[-0.10998 0.33851 -0.16583]  CS2Rot=[1 0 0;0 1 0;0 0 1]  CS3Pos=[-0.078466 0.40468 -0.17639]  CS3Rot=[1 0 0;0 1 0;0 0 1]  CS4Pos=[]  CS4Rot=[]  CS5Pos=[]  CS5Rot=[]  CS6Pos=[]  CS6Rot=[]  CS7Pos=[]  CS7Rot=[]  CS8Pos=[]  CS8Rot=[]  CS9Pos=[]  CS9Rot=[]  CS10Pos=[]  CS10Rot=[]  CS11Pos=[]  CS11Rot=[]  CS12Pos=[]  CS12Rot=[]  CS13Pos=[]  CS13Rot=[]  CS14Pos=[]  CS14Rot=[]  CS15Pos=[]  CS15Rot=[]  CS16Pos=[]  CS16Rot=[]  CS17Pos=[]  CS17Rot=[]  CS18Pos=[]  CS18Rot=[]  CS19Pos=[]  CS19Rot=[]  CS20Pos=[]  CS20Rot=[]
  Tube_Upper-5 : mblibv1/Bodies/Body  DialogController=MECH.DynMechDlgSource  PhysicalDomain=mechanical  SubClassName=Unknown  LeftPortType=workingframe  RightPortType=workingframe  LConnTagsString=CS2  RConnTagsString=CS3  DialogClass=MechanicalBodyBlock  Mass=0.062832  MassUnits=kg  InertiaUnits=kg*m^2  Inertia=[0.00021101 0 0;0 3.1416e-006 0;0 0 0.00021101]  Shape=Cylinder  ShapeDims=[1 1]  ShapeUnits=m  ShapeUse=false  Density=1  DensityUnits=kg/m^3  DensityUse=false  CG=Right$CG$[-0.15591 0.37917 0.028629]$WORLD$WORLD$m$[0.077154 0.28308 -0.95599;-0.34666 0.90664 0.24049;0.93481 0.31284 0.16808]$3x3 Transform$rad$WORLD$  WorkingFrames=Right$CS3$[-0.1276 0.46983 0.059914]$WORLD$WORLD$m$[1 0 0;0 1 0;0 0 1]$3x3 Transform$rad$WORLD$true#Left$CS2$[-0.16697 0.34373 0.0164]$WORLD$WORLD$m$[1 0 0;0 1 0;0 0 1]$3x3 Transform$rad$WORLD$true#Right$CS1$[-0.18422 0.28851 -0.0026554]$WORLD$WORLD$m$[0.077154 0.28308 -0.95599;-0.34666 0.90664 0.24049;0.93481 0.31284 0.16808]$3x3 Transform$rad$WORLD$  CGPos=[-0.15591 0.37917 0.028629]  CGRot=[0.077154 0.28308 -0.95599;-0.34666 0.90664 0.24049;0.93481 0.31284 0.16808]  CS0Pos=[]  CS0Rot=[]  CS1Pos=[-0.18422 0.28851 -0.0026554]  CS1Rot=[0.077154 0.28308 -0.95599;-0.34666 0.90664 0.24049;0.93481 0.31284 0.16808]  CS2Pos=[-0.16697 0.34373 0.0164]  CS2Rot=[1 0 0;0 1 0;0 0 1]  CS3Pos=[-0.1276 0.46983 0.059914]  CS3Rot=[1 0 0;0 1 0;0 0 1]  CS4Pos=[]  CS4Rot=[]  CS5Pos=[]  CS5Rot=[]  CS6Pos=[]  CS6Rot=[]  CS7Pos=[]  CS7Rot=[]  CS8Pos=[]  CS8Rot=[]  CS9Pos=[]  CS9Rot=[]  CS10Pos=[]  CS10Rot=[]  CS11Pos=[]  CS11Rot=[]  CS12Pos=[]  CS12Rot=[]  CS13Pos=[]  CS13Rot=[]  CS14Pos=[]  CS14Rot=[]  CS15Pos=[]  CS15Rot=[]  CS16Pos=[]  CS16Rot=[]  CS17Pos=[]  CS17Rot=[]  CS18Pos=[]  CS18Rot=[]  CS19Pos=[]  CS19Rot=[]  CS20Pos=[]  CS20Rot=[]
  Tube_Upper-6 : mblibv1/Bodies/Body  DialogController=MECH.DynMechDlgSource  PhysicalDomain=mechanical  SubClassName=Unknown  LeftPortType=workingframe  RightPortType=workingframe  LConnTagsString=CS2  RConnTagsString=CS3  DialogClass=MechanicalBodyBlock  Mass=0.062832  MassUnits=kg  InertiaUnits=kg*m^2  Inertia=[0.00021101 0 0;0 3.1416e-006 0;0 0 0.00021101]  Shape=Cylinder  ShapeDims=[1 1]  ShapeUnits=m  ShapeUse=false  Density=1  DensityUnits=kg/m^3  DensityUse=false  CG=Right$CG$[-0.11034 0.38319 0.10677]$WORLD$WORLD$m$[-0.69745 -0.17265 -0.69553;0.2284 0.86638 -0.44409;0.67927 -0.46859 -0.56482]$3x3 Transform$rad$WORLD$  WorkingFrames=Right$CS3$[-0.1276 0.46983 0.059914]$WORLD$WORLD$m$[1 0 0;0 1 0;0 0 1]$3x3 Transform$rad$WORLD$true#Left$CS2$[-0.099263 0.32763 0.13683]$WORLD$WORLD$m$[1 0 0;0 1 0;0 0 1]$3x3 Transform$rad$WORLD$true#Right$CS1$[-0.093072 0.29656 0.15363]$WORLD$WORLD$m$[-0.69745 -0.17265 -0.69553;0.2284 0.86638 -0.44409;0.67927 -0.46859 -0.56482]$3x3 Transform$rad$WORLD$  CGPos=[-0.11034 0.38319 0.10677]  CGRot=[-0.69745 -0.17265 -0.69553;0.2284 0.86638 -0.44409;0.67927 -0.46859 -0.56482]  CS0Pos=[]  CS0Rot=[]  CS1Pos=[-0.093072 0.29656 0.15363]  CS1Rot=[-0.69745 -0.17265 -0.69553;0.2284 0.86638 -0.44409;0.67927 -0.46859 -0.56482]  CS2Pos=[-0.099263 0.32763 0.13683]  CS2Rot=[1 0 0;0 1 0;0 0 1]  CS3Pos=[-0.1276 0.46983 0.059914]  CS3Rot=[1 0 0;0 1 0;0 0 1]  CS4Pos=[]  CS4Rot=[]  CS5Pos=[]  CS5Rot=[]  CS6Pos=[]  CS6Rot=[]  CS7Pos=[]  CS7Rot=[]  CS8Pos=[]  CS8Rot=[]  CS9Pos=[]  CS9Rot=[]  CS10Pos=[]  CS10Rot=[]  CS11Pos=[]  CS11Rot=[]  CS12Pos=[]  CS12Rot=[]  CS13Pos=[]  CS13Rot=[]  CS14Pos=[]  CS14Rot=[]  CS15Pos=[]  CS15Rot=[]  CS16Pos=[]  CS16Rot=[]  CS17Pos=[]  CS17Rot=[]  CS18Pos=[]  CS18Rot=[]  CS19Pos=[]  CS19Rot=[]  CS20Pos=[]  CS20Rot=[]
  Weld : mblibv1/Joints/Weld  DialogController=MECH.DynMechDlgSource  PhysicalDomain=mechanical  SubClassName=Unknown  LeftPortType=blob  RightPortType=blob  LConnTagsString=__newl0  RConnTagsString=__newr0  NumSAPorts=0  CutJoint=off  MarkAsCut=off  Primitives=weld  PrimitiveProps=W$WORLD$[0.57735 0.57735 0.57735]$weld  DialogClass=JointBlock  WAxis=[0.57735 0.57735 0.57735]
  Weld1 : mblibv1/Joints/Weld  DialogController=MECH.DynMechDlgSource  PhysicalDomain=mechanical  SubClassName=Unknown  LeftPortType=blob  RightPortType=blob  LConnTagsString=__newl0  RConnTagsString=__newr0  NumSAPorts=0  CutJoint=off  MarkAsCut=off  Primitives=weld  PrimitiveProps=W$WORLD$[0.57735 0.57735 0.57735]$weld  DialogClass=JointBlock  WAxis=[0.57735 0.57735 0.57735]
  wires:
  [Do] -> Joint Actuator3/1
  [Eo] -> Joint Actuator4/1
  [Fo] -> Joint Actuator5/1
  Joint Sensor1/1 -> [B]
  Joint Sensor2/1 -> [C]
  Joint Sensor3/1 -> [D]
  Joint Sensor4/1 -> [E]
  Joint Sensor5/1 -> [F]
  [A] -> Embedded MATLAB Function/1(i1)
  [B] -> Embedded MATLAB Function/2(i2)
  [C] -> Embedded MATLAB Function/3(i3)
  [D] -> Embedded MATLAB Function/4(i4)
  [E] -> Embedded MATLAB Function/5(i5)
  [F] -> Embedded MATLAB Function/6(i6)
  Embedded MATLAB Function/1(o1) -> [Ao]
  Embedded MATLAB Function/2(o2) -> [Bo]
  Embedded MATLAB Function/3(o3) -> [Co]
  Embedded MATLAB Function/4(o4) -> [Do]
  Embedded MATLAB Function/5(o5) -> [Eo]
  Embedded MATLAB Function/6(o6) -> [Fo]
  [Bo] -> Joint Actuator1/1
  [Co] -> Joint Actuator2/1
  Mux/1 -> Falcon/1, Display4/1
  [Force] -> Gain/1
  Gain/1 -> Saturation/1
  Constant/1 -> Mux/2, Mux/3
  Body Sensor/1 -> Subsystem/1(pos_cur), Current Pos/1
  Body Sensor/2 -> Subsystem/3(velocity)
  Falcon/1 -> Map2Plat/1, Demux/1
  Subsystem/1(F_Out1) -> [Force], Force disp/1
  [pos_new] -> Subsystem/2(pos_new)
  Demux/2 -> Mux1/2
  Demux/3 -> Mux1/3
  Map2Plat/1 -> Mux1/1
  Mux1/1 -> [pos_new], Display2/1
  Saturation/1 -> Demux1/1
  [Force] -> Demux2/1
  Demux2/2 -> Embedded MATLAB Function/7(f)
  Demux1/2 -> Mux/1
  connections:
  Weld/LConn1 -- RootPart/RConn1
  Weld/RConn1 -- Base-1/LConn1
  Spherical/RConn1 -- Tube_Base-5/LConn1
  Cylindrical/LConn1 -- Tube_Base-5/RConn1
  Cylindrical/RConn1 -- Tube_Upper-5/LConn1
  Cylindrical1/LConn1 -- Tube_Base-4/RConn1
  Cylindrical1/RConn1 -- Tube_Upper-6/LConn1
  Spherical2/LConn1 -- Base-1/RConn5
  Spherical2/RConn1 -- Tube_Base-1/LConn1
  Cylindrical2/LConn1 -- Tube_Base-1/RConn1
  Cylindrical2/RConn1 -- Tube_Upper-1/LConn1
  Spherical3/LConn1 -- Base-1/RConn3
  Spherical3/RConn1 -- Tube_Base-3/LConn1
  Spherical4/LConn1 -- Base-1/RConn1
  Spherical4/RConn1 -- Tube_Base-2/LConn1
  Cylindrical3/LConn1 -- Tube_Base-3/RConn1
  Cylindrical3/RConn1 -- Tube_Upper-3/LConn1
  Spherical5/LConn1 -- Tube_Upper-3/RConn1
  Spherical5/RConn1 -- Plate-1/LConn3
  Spherical6/LConn1 -- Tube_Upper-1/RConn1
  Spherical6/RConn1 -- Plate-1/LConn5
  Cylindrical4/RConn1 -- Tube_Upper-2/LConn1
  Spherical8/LConn1 -- Tube_Upper-2/RConn1
  Spherical8/RConn1 -- Plate-1/LConn2
  Subsystem1/RConn1 -- Plate-1/LConn1
  Spherical10/LConn1 -- Tube_Upper-5/RConn1
  Spherical10/RConn1 -- Plate-1/LConn4
  Spherical11/LConn1 -- Tube_Upper-6/RConn1
  Spherical11/RConn1 -- Plate-1/LConn6
  Weld1/LConn1 -- RootGround/RConn1
  Weld1/RConn1 -- RootPart/LConn1
  RootGround/LConn1 -- Machine Environment/RConn1
  Spherical1/RConn1 -- Tube_Base-4/LConn1
  Base-1/RConn6 -- Spherical1/LConn1
  Base-1/RConn4 -- Spherical/LConn1
  Tube_Base-2/RConn1 -- Cylindrical4/LConn1
  Base-1/RConn2 -- Subsystem1/LConn1
  Joint Actuator1/RConn1 -- Cylindrical4/LConn2
  Joint Actuator2/RConn1 -- Cylindrical3/LConn2
  Joint Actuator3/RConn1 -- Cylindrical/LConn2
  Joint Actuator4/RConn1 -- Cylindrical2/LConn2
  Joint Actuator5/RConn1 -- Cylindrical1/LConn2
  Cylindrical4/RConn2 -- Joint Sensor1/LConn1
  Cylindrical3/RConn2 -- Joint Sensor2/LConn1
  Cylindrical/RConn2 -- Joint Sensor3/LConn1
  Cylindrical2/RConn2 -- Joint Sensor4/LConn1
  Cylindrical1/RConn2 -- Joint Sensor5/LConn1
  Plate-1/RConn1 -- Body Sensor/LConn1

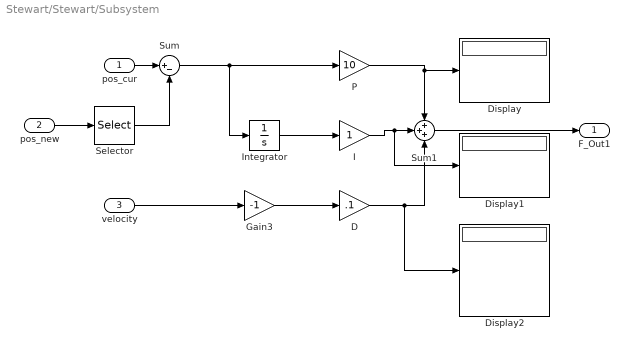
== system Stewart/Stewart/Subsystem ==
  pos_cur : Inport
  pos_new : Inport  Port=2
  velocity : Inport  Port=3
  D : Gain  Gain=.1  ParameterDataType=sfix(16)  ParameterScaling=2^0  OutDataType=sfix(16)  OutScaling=2^0
  Display : Display
  Display1 : Display
  Display2 : Display
  Gain3 : Gain  Gain=-1  ParameterDataType=sfix(16)  ParameterScaling=2^0  OutDataType=sfix(16)  OutScaling=2^0
  I : Gain  ParameterDataType=sfix(16)  ParameterScaling=2^0  OutDataType=sfix(16)  OutScaling=2^0
  Integrator : Integrator
  P : Gain  Gain=10  ParameterDataType=sfix(16)  ParameterScaling=2^0  OutDataType=sfix(16)  OutScaling=2^0
  Selector : Selector  InputPortWidth=3  IndexOptions=Index vector (dialog)  Indices=[3 1 2]  OutputSizes=1
  Sum : Sum  Inputs=|+-  OutDataType=sfix(16)  OutScaling=2^0
  Sum1 : Sum  Inputs=+++  OutDataType=sfix(16)  OutScaling=2^0
  F_Out1 : Outport
  wires:
  pos_cur/1 -> Sum/1
  pos_new/1 -> Selector/1
  Sum/1 -> P/1, Integrator/1
  Integrator/1 -> I/1
  velocity/1 -> Gain3/1
  Gain3/1 -> D/1
  P/1 -> Sum1/1, Display/1
  I/1 -> Sum1/2, Display1/1
  D/1 -> Sum1/3, Display2/1
  Sum1/1 -> F_Out1/1
  Selector/1 -> Sum/2

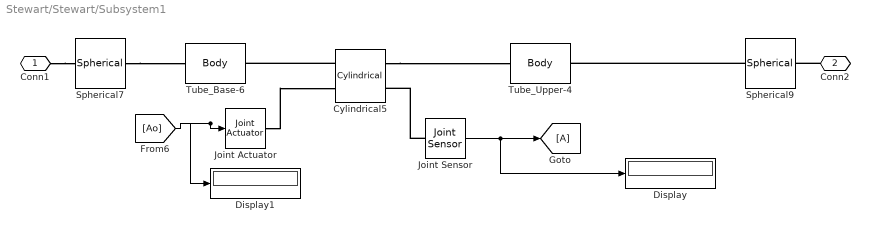
== system Stewart/Stewart/Subsystem1 ==
  Cylindrical5 : mblibv1/Joints/Cylindrical  DialogController=MECH.DynMechDlgSource  PhysicalDomain=mechanical  SubClassName=Unknown  LeftPortType=blob  RightPortType=blob  LConnTagsString=__newl0|SA1  RConnTagsString=__newr0|SA1  NumSAPorts=2  CutJoint=off  MarkAsCut=off  Primitives=prismatic  PrimitiveProps=P1$World$[0.57086 -0.81077 0.12949]$prismatic#R1$World$[0.57086 -0.81077 0.12949]$revolute  DialogClass=JointBlock  P1Axis=[0.57086 -0.81077 0.12949]  R1Axis=[0.57086 -0.81077 0.12949]
  Display : Display
  Display1 : Display
  Joint Actuator : mblibv1/Sensors &  Actuators/Joint Actuator  DialogController=MECH.DynMechDlgSource  SystemSampleTime=-1  PhysicalDomain=Mechanical  PortType=blob  ActuationStyle=Force  AngleUnits=deg  ArcVelocityUnits=deg/s  ArcAccelerationUnits=deg/s^2  CoordPositionUnits=m  VelocityUnits=m/s  AccelerationUnits=m/s^2  ForceUnits=N  TorqueUnits=N*m  ActiveIO=on  Width=1  DialogClass=MechanicalActuatorBlock  Primitive=P1  ReferenceFrame=Absolute (World)
  Joint Sensor : mblibv1/Sensors &  Actuators/Joint Sensor  DialogController=MECH.DynMechDlgSource  SystemSampleTime=-1  PhysicalDomain=Mechanical  PortType=blob  Muxed=on  Pose=off  Angle=on  AngleUnits=deg  ArcVelocity=off  ArcVelocityUnits=deg/s  ArcAcceleration=off  ArcAccelerationUnits=deg/s^2  CoordPosition=on  CoordPositionUnits=m  Velocity=off  VelocityUnits=m/s  Acceleration=off  AccelerationUnits=m/s^2  Quaternion=on  QuaternionDT=off  QuaternionDDT=off  QuaternionUnits=off  OutputVector=[1]  ActiveIO=on  Width=1  DialogClass=MechanicalSensorBlock  Primitive=P1  Force=off  ForceUnits=N  Torque=off  TorqueUnits=N-m  ReferenceFrame=Absolute (World)  ReactionSensedSide=Base  ReactionReferenceFrame=Absolute (World)  ReactionForce=off  ReactionForceUnits=N  ReactionMoment=off  ReactionMomentUnits=N-m
  Spherical7 : mblibv1/Joints/Spherical  DialogController=MECH.DynMechDlgSource  PhysicalDomain=mechanical  SubClassName=Unknown  LeftPortType=blob  RightPortType=blob  LConnTagsString=__newl0  RConnTagsString=__newr0  NumSAPorts=0  CutJoint=off  MarkAsCut=off  Primitives=spherical  PrimitiveProps=S$WORLD$[0 0 0]$spherical  DialogClass=JointBlock  SAxis=[0 0 0]
  Spherical9 : mblibv1/Joints/Spherical  DialogController=MECH.DynMechDlgSource  PhysicalDomain=mechanical  SubClassName=Unknown  LeftPortType=blob  RightPortType=blob  LConnTagsString=__newl0  RConnTagsString=__newr0  NumSAPorts=0  CutJoint=off  MarkAsCut=off  Primitives=spherical  PrimitiveProps=S$WORLD$[0 0 0]$spherical  DialogClass=JointBlock  SAxis=[0 0 0]
  Tube_Base-6 : mblibv1/Bodies/Body  DialogController=MECH.DynMechDlgSource  PhysicalDomain=mechanical  SubClassName=Unknown  LeftPortType=workingframe  RightPortType=workingframe  LConnTagsString=CS2  RConnTagsString=CS3  DialogClass=MechanicalBodyBlock  Mass=0.12566  MassUnits=kg  InertiaUnits=kg*m^2  Inertia=[0.0016787 0 0;0 6.2832e-006 0;0 0 0.0016787]  Shape=Cylinder  ShapeDims=[1 1]  ShapeUnits=m  ShapeUse=false  Density=1  DensityUnits=kg/m^3  DensityUse=false  CG=Right$CG$[0.10562 0.14323 -0.13464]$WORLD$WORLD$m$[0.81852 -0.57086 0.064337;0.54963 0.81077 0.2014;-0.16713 -0.12949 0.97739]$3x3 Transform$rad$WORLD$  WorkingFrames=Left$CS2$[0.2198 -0.018929 -0.10874]$WORLD$WORLD$m$[1 0 0;0 1 0;0 0 1]$3x3 Transform$rad$WORLD$true#Right$CS3$[-0.0085488 0.30538 -0.16053]$WORLD$WORLD$m$[1 0 0;0 1 0;0 0 1]$3x3 Transform$rad$WORLD$true#Right$CS1$[0.2198 -0.018929 -0.10874]$WORLD$WORLD$m$[0.81852 -0.57086 0.064337;0.54963 0.81077 0.2014;-0.16713 -0.12949 0.97739]$3x3 Transform$rad$WORLD$  CGPos=[0.10562 0.14323 -0.13464]  CGRot=[0.81852 -0.57086 0.064337;0.54963 0.81077 0.2014;-0.16713 -0.12949 0.97739]  CS0Pos=[]  CS0Rot=[]  CS1Pos=[0.2198 -0.018929 -0.10874]  CS1Rot=[0.81852 -0.57086 0.064337;0.54963 0.81077 0.2014;-0.16713 -0.12949 0.97739]  CS2Pos=[0.2198 -0.018929 -0.10874]  CS2Rot=[1 0 0;0 1 0;0 0 1]  CS3Pos=[-0.0085488 0.30538 -0.16053]  CS3Rot=[1 0 0;0 1 0;0 0 1]  CS4Pos=[]  CS4Rot=[]  CS5Pos=[]  CS5Rot=[]  CS6Pos=[]  CS6Rot=[]  CS7Pos=[]  CS7Rot=[]  CS8Pos=[]  CS8Rot=[]  CS9Pos=[]  CS9Rot=[]  CS10Pos=[]  CS10Rot=[]  CS11Pos=[]  CS11Rot=[]  CS12Pos=[]  CS12Rot=[]  CS13Pos=[]  CS13Rot=[]  CS14Pos=[]  CS14Rot=[]  CS15Pos=[]  CS15Rot=[]  CS16Pos=[]  CS16Rot=[]  CS17Pos=[]  CS17Rot=[]  CS18Pos=[]  CS18Rot=[]  CS19Pos=[]  CS19Rot=[]  CS20Pos=[]  CS20Rot=[]
  Tube_Upper-4 : mblibv1/Bodies/Body  DialogController=MECH.DynMechDlgSource  PhysicalDomain=mechanical  SubClassName=Unknown  LeftPortType=workingframe  RightPortType=workingframe  LConnTagsString=CS2  RConnTagsString=CS3  DialogClass=MechanicalBodyBlock  Mass=0.062832  MassUnits=kg  InertiaUnits=kg*m^2  Inertia=[0.00021101 0 0;0 3.1416e-006 0;0 0 0.00021101]  Shape=Cylinder  ShapeDims=[1 1]  ShapeUnits=m  ShapeUse=false  Density=1  DensityUnits=kg/m^3  DensityUse=false  CG=Right$CG$[-0.021379 0.3236 -0.16344]$WORLD$WORLD$m$[0.0027197 -0.57086 0.82104;-0.15584 0.81077 0.56424;-0.98778 -0.12949 -0.08676]$3x3 Transform$rad$WORLD$  WorkingFrames=Left$CS2$[-0.0085488 0.30538 -0.16053]$WORLD$WORLD$m$[1 0 0;0 1 0;0 0 1]$3x3 Transform$rad$WORLD$true#Right$CS3$[-0.078466 0.40468 -0.17639]$WORLD$WORLD$m$[1 0 0;0 1 0;0 0 1]$3x3 Transform$rad$WORLD$true#Right$CS1$[0.035707 0.24253 -0.15049]$WORLD$WORLD$m$[0.0027197 -0.57086 0.82104;-0.15584 0.81077 0.56424;-0.98778 -0.12949 -0.08676]$3x3 Transform$rad$WORLD$  CGPos=[-0.021379 0.3236 -0.16344]  CGRot=[0.0027197 -0.57086 0.82104;-0.15584 0.81077 0.56424;-0.98778 -0.12949 -0.08676]  CS0Pos=[]  CS0Rot=[]  CS1Pos=[0.035707 0.24253 -0.15049]  CS1Rot=[0.0027197 -0.57086 0.82104;-0.15584 0.81077 0.56424;-0.98778 -0.12949 -0.08676]  CS2Pos=[-0.0085488 0.30538 -0.16053]  CS2Rot=[1 0 0;0 1 0;0 0 1]  CS3Pos=[-0.078466 0.40468 -0.17639]  CS3Rot=[1 0 0;0 1 0;0 0 1]  CS4Pos=[]  CS4Rot=[]  CS5Pos=[]  CS5Rot=[]  CS6Pos=[]  CS6Rot=[]  CS7Pos=[]  CS7Rot=[]  CS8Pos=[]  CS8Rot=[]  CS9Pos=[]  CS9Rot=[]  CS10Pos=[]  CS10Rot=[]  CS11Pos=[]  CS11Rot=[]  CS12Pos=[]  CS12Rot=[]  CS13Pos=[]  CS13Rot=[]  CS14Pos=[]  CS14Rot=[]  CS15Pos=[]  CS15Rot=[]  CS16Pos=[]  CS16Rot=[]  CS17Pos=[]  CS17Rot=[]  CS18Pos=[]  CS18Rot=[]  CS19Pos=[]  CS19Rot=[]  CS20Pos=[]  CS20Rot=[]
  Conn1 : PMIOPort  Port=1  Side=Left
  Conn2 : PMIOPort  Orientation=left  Port=2  Side=Right
  wires:
  Joint Sensor/1 -> Display/1, [A]
  [Ao] -> Joint Actuator/1, Display1/1
  connections:
  Cylindrical5/LConn1 -- Tube_Base-6/RConn1
  Joint Actuator/RConn1 -- Cylindrical5/LConn2
  Cylindrical5/RConn1 -- Tube_Upper-4/LConn1
  Joint Sensor/LConn1 -- Cylindrical5/RConn2
  Spherical7/RConn1 -- Tube_Base-6/LConn1
  Spherical9/LConn1 -- Tube_Upper-4/RConn1
  Conn1/RConn1 -- Spherical7/LConn1
  Conn2/RConn1 -- Spherical9/RConn1

== matlab function Stewart/Embedded MATLAB Function ==
  data: i1 input inherited; o1 output inherited; i2 input inherited; i3 input inherited; i4 input inherited; i5 input inherited; i6 input inherited; o2 output inherited; o3 output inherited; o4 output inherited; o5 output inherited; o6 output inherited; f input inherited
function [o1, o2, o3, o4, o5, o6] = fcn(i1, i2, i3, i4, i5, i6, f)
% This block supports the Embedded MATLAB subset.
% See the help menu for details. 


force = f;

if i1 > -.1
    o1=force;
    o2=force;
    o3=force;
    o4=force;
    o5=force;
    o6=force;
else
    o1=0;
    o2=0;
    o3=0;
    o4=0;
    o5=0;
    o6=0;
end
